simulink model "Appl_PowerMangeModel"  (R2018b)
settings: configuration reference "CodeConfig_10_ms" (kept outside this file)
undefined symbols (not defined in the file): CAL_DownVolt_600ms, CAL_Filiter_500ms, CAL_UpVolt_200ms, D_POWER_ADJUST_15800MV, D_POWER_ADJUST_7800MV, D_POWER_HIGH_DN, D_POWER_HIGH_UP, D_POWER_Invalid, D_POWER_LOW_DN, D_POWER_LOW_UP, D_POWER_NORMAL_DN, D_POWER_NORMAL_UP, D_POWER_OVER_DN, D_POWER_STOP_UP, enPowerModeSts, FALSE, TRUE
libraries: DareLib x7, simulink x5
settings Model: Creator=Administrator  LastModifiedBy=Administrator
settings ConfigSetRef: SourceLocation=Base Workspace

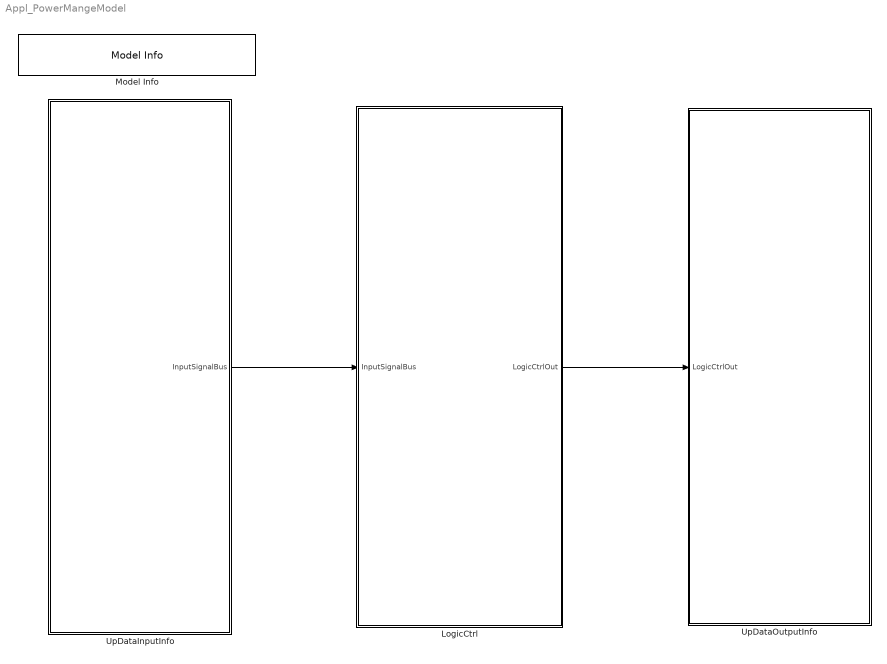
== system Appl_PowerMangeModel ==
  LogicCtrl : Subsystem  Priority=2  TreatAsAtomicUnit=on
      settings: RTWSystemCode=Nonreusable function  RTWFcnNameOpts=Use subsystem name
  Model Info : simulink/Model-Wide Utilities/Model Info  Frame=on  DisplayStringWithTags=Version：%<ModelVersion>  HorizontalTextAlignment=Center  LeftAlignmentValue=0.5
  UpDataInputInfo : Subsystem  Priority=1  TreatAsAtomicUnit=on
      settings: RTWSystemCode=Nonreusable function  RTWFcnNameOpts=Use subsystem name
  UpDataOutputInfo : Subsystem  Priority=3  TreatAsAtomicUnit=on
      settings: RTWSystemCode=Nonreusable function  RTWFcnNameOpts=Use subsystem name
  wires:
  UpDataInputInfo/1(InputSignalBus) -> LogicCtrl/1(InputSignalBus)
  LogicCtrl/1(LogicCtrlOut) -> UpDataOutputInfo/1(LogicCtrlOut)

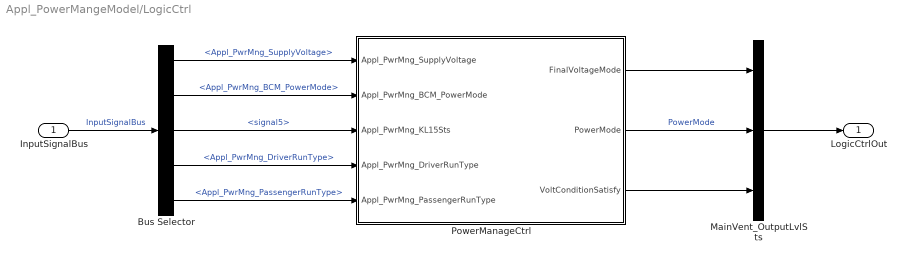
== system Appl_PowerMangeModel/LogicCtrl ==
  InputSignalBus : Inport
  Bus Selector : BusSelector  OutputSignals=Rte_SignalBus.Appl_PwrMng_SupplyVoltage,Rte_SignalBus.Appl_PwrMng_BCM_PowerMode,Rte_SignalBus.signal5,Rte_SignalBus.Appl_PwrMng_DriverRunType,Rte_SignalBus.Appl_PwrMng_PassengerRunType
  MainVent_OutputLvlSts : BusCreator  Inputs=3
  PowerManageCtrl : Subsystem  Description=电源管理逻辑处理
      settings: AttributesFormatString=%<Description>
  LogicCtrlOut : Outport
  wires:
  InputSignalBus/1 -> Bus Selector/1  "InputSignalBus"
  MainVent_OutputLvlSts/1 -> LogicCtrlOut/1
  PowerManageCtrl/1(FinalVoltageMode) -> MainVent_OutputLvlSts/1
  Bus Selector/2 -> PowerManageCtrl/2(Appl_PwrMng_BCM_PowerMode)  "<Appl_PwrMng_BCM_PowerMode>"
  Bus Selector/1 -> PowerManageCtrl/1(Appl_PwrMng_SupplyVoltage)  "<Appl_PwrMng_SupplyVoltage>"
  Bus Selector/3 -> PowerManageCtrl/3(Appl_PwrMng_KL15Sts)  "<signal5>"
  PowerManageCtrl/2(PowerMode) -> MainVent_OutputLvlSts/2  "PowerMode"
  Bus Selector/4 -> PowerManageCtrl/4(Appl_PwrMng_DriverRunType)  "<Appl_PwrMng_DriverRunType>"
  Bus Selector/5 -> PowerManageCtrl/5(Appl_PwrMng_PassengerRunType)  "<Appl_PwrMng_PassengerRunType>"
  PowerManageCtrl/3(VoltConditionSatisfy) -> MainVent_OutputLvlSts/3

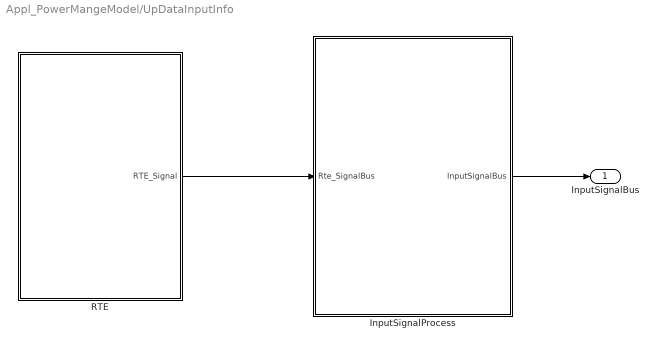
== system Appl_PowerMangeModel/UpDataInputInfo ==
  InputSignalProcess : Subsystem  Description=数据处理
      settings: AttributesFormatString=%<Description>  RTWSystemCode=Nonreusable function  RTWFcnNameOpts=Use subsystem name
  RTE : Subsystem  Description=接口自动生成  TreatAsAtomicUnit=on
      settings: AttributesFormatString=%<Description>  RTWSystemCode=Nonreusable function  RTWFcnNameOpts=Use subsystem name
  InputSignalBus : Outport
  wires:
  RTE/1(RTE_Signal) -> InputSignalProcess/1(Rte_SignalBus)
  InputSignalProcess/1(InputSignalBus) -> InputSignalBus/1

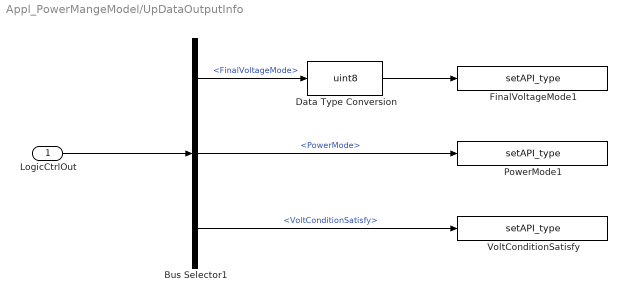
== system Appl_PowerMangeModel/UpDataOutputInfo ==
  LogicCtrlOut : Inport
  Bus Selector1 : BusSelector  OutputSignals=FinalVoltageMode,PowerMode,VoltConditionSatisfy
  Data Type Conversion : DataTypeConversion  OutDataTypeStr=uint8
  FinalVoltageMode1 : DareLib/Dare/setAPI_type  g_funcname=Rte_SetVfb_VoltMode  g_type=uint8  g_size=-1
      settings: AttributesFormatString=%<g_funcname>  SourceProductName=Dare Library
  PowerMode1 : DareLib/Dare/setAPI_type  g_funcname=Rte_SetVfb_PowerMode  g_type=uint8  g_size=-1
      settings: AttributesFormatString=%<g_funcname>  SourceProductName=Dare Library
  VoltConditionSatisfy : DareLib/Dare/setAPI_type  g_funcname=Rte_SetVfb_VoltSatisfy  g_type=uint8  g_size=-1
      settings: AttributesFormatString=%<g_funcname>  SourceProductName=Dare Library
  wires:
  LogicCtrlOut/1 -> Bus Selector1/1
  Bus Selector1/1 -> Data Type Conversion/1  "<FinalVoltageMode>"
  Bus Selector1/2 -> PowerMode1/1  "<PowerMode>"
  Data Type Conversion/1 -> FinalVoltageMode1/1
  Bus Selector1/3 -> VoltConditionSatisfy/1  "<VoltConditionSatisfy>"

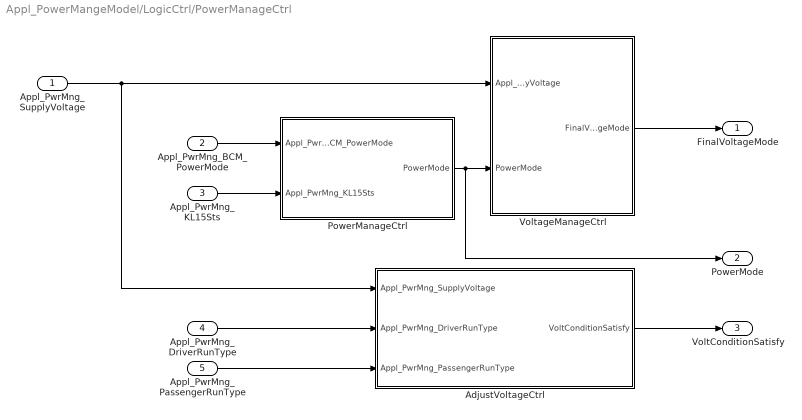
== system Appl_PowerMangeModel/LogicCtrl/PowerManageCtrl ==
  Appl_PwrMng_SupplyVoltage : Inport
  Appl_PwrMng_BCM_PowerMode : Inport  Port=2
  Appl_PwrMng_KL15Sts : Inport  Port=3
  Appl_PwrMng_DriverRunType : Inport  Port=4
  Appl_PwrMng_PassengerRunType : Inport  Port=5
  AdjustVoltageCtrl : Subsystem  Description=调节电机电压控制
      settings: AttributesFormatString=%<Description>
  PowerManageCtrl : Subsystem  Description=系统电源模式管理
      settings: AttributesFormatString=%<Description>
  VoltageManageCtrl : Subsystem  Description=电压模式切换
      settings: AttributesFormatString=%<Description>
  FinalVoltageMode : Outport
  PowerMode : Outport  Port=2
  VoltConditionSatisfy : Outport  Port=3
  wires:
  VoltageManageCtrl/1(FinalVoltageMode) -> FinalVoltageMode/1
  Appl_PwrMng_SupplyVoltage/1 -> AdjustVoltageCtrl/1(Appl_PwrMng_SupplyVoltage), VoltageManageCtrl/1(Appl_PwrMng_SupplyVoltage)
  Appl_PwrMng_KL15Sts/1 -> PowerManageCtrl/2(Appl_PwrMng_KL15Sts)
  PowerManageCtrl/1(PowerMode) -> PowerMode/1, VoltageManageCtrl/2(PowerMode)
  Appl_PwrMng_BCM_PowerMode/1 -> PowerManageCtrl/1(Appl_PwrMng_BCM_PowerMode)
  Appl_PwrMng_DriverRunType/1 -> AdjustVoltageCtrl/2(Appl_PwrMng_DriverRunType)
  Appl_PwrMng_PassengerRunType/1 -> AdjustVoltageCtrl/3(Appl_PwrMng_PassengerRunType)
  AdjustVoltageCtrl/1(VoltConditionSatisfy) -> VoltConditionSatisfy/1

== system Appl_PowerMangeModel/UpDataInputInfo/InputSignalProcess ==
  Rte_SignalBus : Inport
  Bus Creator : BusCreator  Inputs=1
  InputSignalBus : Outport
  wires:
  Bus Creator/1 -> InputSignalBus/1
  Rte_SignalBus/1 -> Bus Creator/1  "Rte_SignalBus"

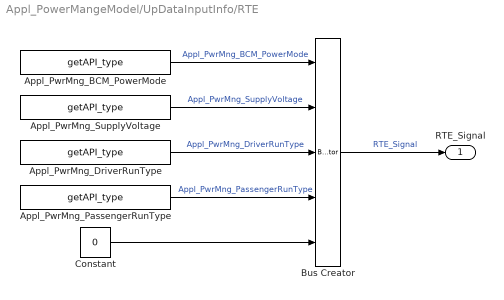
== system Appl_PowerMangeModel/UpDataInputInfo/RTE ==
  Appl_PwrMng_BCM_PowerMode : DareLib/Dare/getAPI_type  g_funcname=CanRx_0x283_BDC_PDU  g_param=""  g_type=uint8  g_size=-1
      settings: AttributesFormatString=%<g_funcname>  SourceProductName=Dare Library
  Appl_PwrMng_DriverRunType : DareLib/Dare/getAPI_type  g_funcname=Rte_GetVfb_DrMoveType  g_param=""  g_type=uint8  g_enum=enSeatMotorRunTye  g_size=-1
      settings: AttributesFormatString=%<g_funcname>  SourceProductName=Dare Library
  Appl_PwrMng_PassengerRunType : DareLib/Dare/getAPI_type  g_funcname=Rte_GetVfb_PaMoveType  g_param=""  g_type=uint8  g_enum=enSeatMotorRunTye  g_size=-1
      settings: AttributesFormatString=%<g_funcname>  SourceProductName=Dare Library
  Appl_PwrMng_SupplyVoltage : DareLib/Dare/getAPI_type  g_funcname=Srvl_Get_SupplyVoltage  g_param=""  g_type=uint16  g_size=-1
      settings: AttributesFormatString=%<g_funcname>  SourceProductName=Dare Library
  Bus Creator : BusCreator  Inputs=5
  Constant : Constant  Value=0  OutDataTypeStr=uint8
  RTE_Signal : Outport
  wires:
  Bus Creator/1 -> RTE_Signal/1  "RTE_Signal"
  Appl_PwrMng_BCM_PowerMode/1 -> Bus Creator/1  "Appl_PwrMng_BCM_PowerMode"
  Appl_PwrMng_SupplyVoltage/1 -> Bus Creator/2  "Appl_PwrMng_SupplyVoltage"
  Appl_PwrMng_DriverRunType/1 -> Bus Creator/3  "Appl_PwrMng_DriverRunType"
  Appl_PwrMng_PassengerRunType/1 -> Bus Creator/4  "Appl_PwrMng_PassengerRunType"
  Constant/1 -> Bus Creator/5

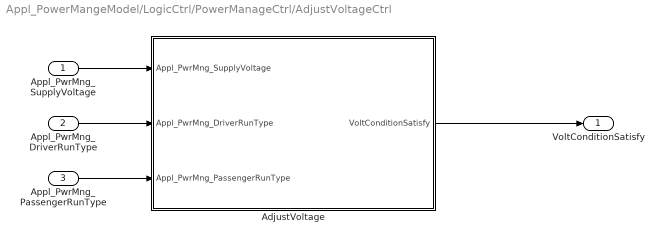
== system Appl_PowerMangeModel/LogicCtrl/PowerManageCtrl/AdjustVoltageCtrl ==
  Appl_PwrMng_SupplyVoltage : Inport
  Appl_PwrMng_DriverRunType : Inport  Port=2
  Appl_PwrMng_PassengerRunType : Inport  Port=3
  AdjustVoltage : Stateflow chart  TreatAsAtomicUnit=on
  VoltConditionSatisfy : Outport
  wires:
  Appl_PwrMng_SupplyVoltage/1 -> AdjustVoltage/1(Appl_PwrMng_SupplyVoltage)
  AdjustVoltage/1(VoltConditionSatisfy) -> VoltConditionSatisfy/1
  Appl_PwrMng_DriverRunType/1 -> AdjustVoltage/2(Appl_PwrMng_DriverRunType)
  Appl_PwrMng_PassengerRunType/1 -> AdjustVoltage/3(Appl_PwrMng_PassengerRunType)

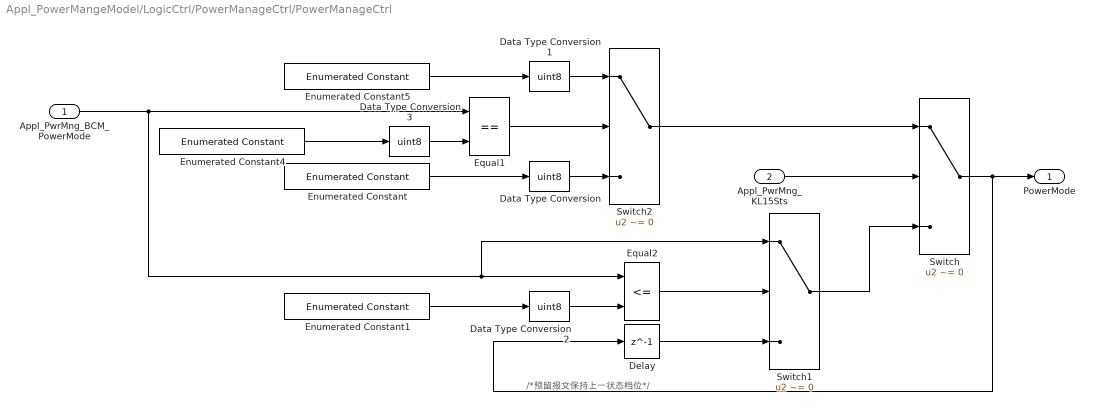
== system Appl_PowerMangeModel/LogicCtrl/PowerManageCtrl/PowerManageCtrl ==
  note: /*预留报文保持上一状态档位*/
  Appl_PwrMng_BCM_PowerMode : Inport
  Appl_PwrMng_KL15Sts : Inport  Port=2
  Data Type Conversion{,1..3} (4 alike) : DataTypeConversion  OutDataTypeStr=uint8
  Delay : Delay  DelayLength=1  InitialCondition=0  InputProcessing=Inherited
  Enumerated Constant : simulink/Sources/Enumerated Constant  OutDataTypeStr=Enum: enPowerModeSts  Value=enPowerModeSts.EN_ON  SampleTime=inf
      settings: SourceProductName=Simulink
  Enumerated Constant1 : simulink/Sources/Enumerated Constant  OutDataTypeStr=Enum: enPowerModeSts  Value=enPowerModeSts.EN_CRANK  SampleTime=inf
      settings: SourceProductName=Simulink
  Enumerated Constant4 : simulink/Sources/Enumerated Constant  OutDataTypeStr=Enum: enPowerModeSts  Value=enPowerModeSts.EN_CRANK  SampleTime=inf
      settings: SourceProductName=Simulink
  Enumerated Constant5 : simulink/Sources/Enumerated Constant  OutDataTypeStr=Enum: enPowerModeSts  Value=enPowerModeSts.EN_CRANK  SampleTime=inf
      settings: SourceProductName=Simulink
  Equal1 : RelationalOperator  Operator===  OutDataTypeStr=boolean  RndMeth=Simplest
  Equal2 : RelationalOperator  Operator=<=  OutDataTypeStr=boolean  RndMeth=Simplest
  Switch : Switch  Criteria=u2 ~= 0
  Switch1 : Switch  Criteria=u2 ~= 0  OutDataTypeStr=uint8
  Switch2 : Switch  Criteria=u2 ~= 0  OutDataTypeStr=uint8
  PowerMode : Outport
  wires:
  Appl_PwrMng_KL15Sts/1 -> Switch/2
  Enumerated Constant/1 -> Data Type Conversion/1
  Enumerated Constant4/1 -> Data Type Conversion3/1
  Equal1/1 -> Switch2/2
  Enumerated Constant5/1 -> Data Type Conversion1/1
  Switch2/1 -> Switch/1
  Enumerated Constant1/1 -> Data Type Conversion2/1
  Appl_PwrMng_BCM_PowerMode/1 -> Switch1/1, Equal2/1, Equal1/1
  Equal2/1 -> Switch1/2
  Switch1/1 -> Switch/3
  Delay/1 -> Switch1/3
  Switch/1 -> Delay/1, PowerMode/1
  Data Type Conversion/1 -> Switch2/3
  Data Type Conversion1/1 -> Switch2/1
  Data Type Conversion2/1 -> Equal2/2
  Data Type Conversion3/1 -> Equal1/2

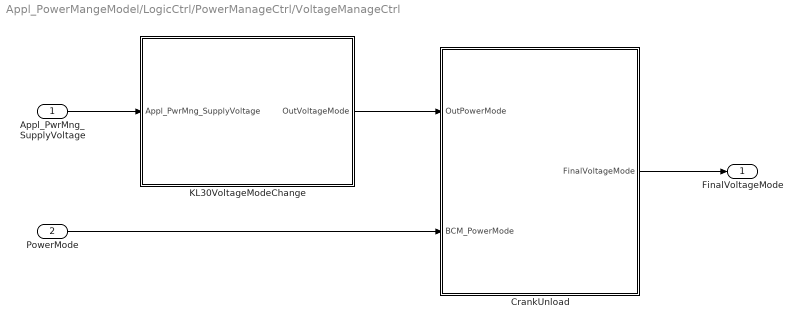
== system Appl_PowerMangeModel/LogicCtrl/PowerManageCtrl/VoltageManageCtrl ==
  Appl_PwrMng_SupplyVoltage : Inport
  PowerMode : Inport  Port=2
  CrankUnload : Stateflow chart  TreatAsAtomicUnit=on
  KL30VoltageModeChange : Stateflow chart  TreatAsAtomicUnit=on
  FinalVoltageMode : Outport
  wires:
  CrankUnload/1(FinalVoltageMode) -> FinalVoltageMode/1
  Appl_PwrMng_SupplyVoltage/1 -> KL30VoltageModeChange/1(Appl_PwrMng_SupplyVoltage)
  PowerMode/1 -> CrankUnload/2(BCM_PowerMode)
  KL30VoltageModeChange/1(OutVoltageMode) -> CrankUnload/1(OutPowerMode)

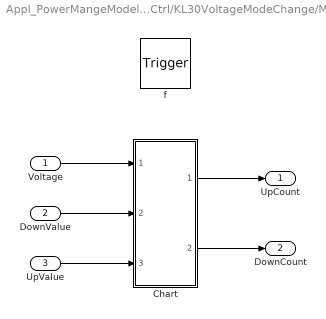
== system Appl_PowerMangeModel/LogicCtrl/PowerManageCtrl/VoltageManageCtrl/KL30VoltageModeChange/ModeChangeFunction ==
  Voltage : Inport  OutDataTypeStr=uint16
  DownValue : Inport  Port=2  OutDataTypeStr=uint16
  UpValue : Inport  Port=3  OutDataTypeStr=uint16
  f : TriggerPort  TriggerType=function-call  VariantControl=(inherit)
      settings: CopyFcn=Stateflow.SLINSF.SimulinkMan.removeBlockPreDeleteFcn  PreDeleteFcn=Stateflow.SLINSF.SimulinkMan.unsafePredeleteFcn
  Chart : Stateflow chart  TreatAsAtomicUnit=on
  UpCount : Outport
  DownCount : Outport  Port=2
  wires:
  Voltage/1 -> Chart/1(Voltage)
  DownValue/1 -> Chart/2(DownValue)
  Chart/1(UpCount) -> UpCount/1
  UpValue/1 -> Chart/3(UpValue)
  Chart/2(DownCount) -> DownCount/1

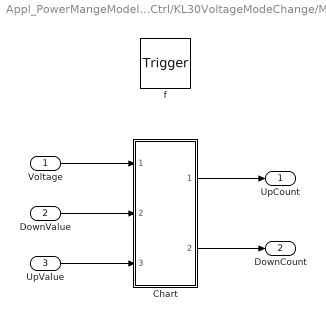
== system Appl_PowerMangeModel/LogicCtrl/PowerManageCtrl/VoltageManageCtrl/KL30VoltageModeChange/ModeChangeFunction1 ==
  Voltage : Inport  OutDataTypeStr=uint16
  DownValue : Inport  Port=2  OutDataTypeStr=uint16
  UpValue : Inport  Port=3  OutDataTypeStr=uint16
  f : TriggerPort  TriggerType=function-call  VariantControl=(inherit)
      settings: CopyFcn=Stateflow.SLINSF.SimulinkMan.removeBlockPreDeleteFcn  PreDeleteFcn=Stateflow.SLINSF.SimulinkMan.unsafePredeleteFcn
  Chart : Stateflow chart  TreatAsAtomicUnit=on
  UpCount : Outport
  DownCount : Outport  Port=2
  wires:
  Voltage/1 -> Chart/1(Voltage)
  DownValue/1 -> Chart/2(DownValue)
  Chart/1(UpCount) -> UpCount/1
  UpValue/1 -> Chart/3(UpValue)
  Chart/2(DownCount) -> DownCount/1

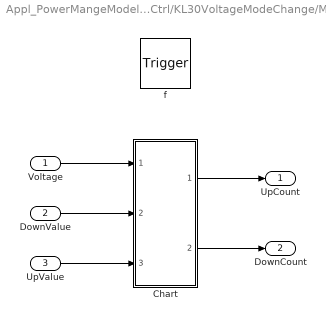
== system Appl_PowerMangeModel/LogicCtrl/PowerManageCtrl/VoltageManageCtrl/KL30VoltageModeChange/ModeChangeFunction2 ==
  Voltage : Inport  OutDataTypeStr=uint16
  DownValue : Inport  Port=2  OutDataTypeStr=uint16
  UpValue : Inport  Port=3  OutDataTypeStr=uint16
  f : TriggerPort  TriggerType=function-call  VariantControl=(inherit)
      settings: CopyFcn=Stateflow.SLINSF.SimulinkMan.removeBlockPreDeleteFcn  PreDeleteFcn=Stateflow.SLINSF.SimulinkMan.unsafePredeleteFcn
  Chart : Stateflow chart  TreatAsAtomicUnit=on
  UpCount : Outport
  DownCount : Outport  Port=2
  wires:
  Voltage/1 -> Chart/1(Voltage)
  DownValue/1 -> Chart/2(DownValue)
  Chart/1(UpCount) -> UpCount/1
  UpValue/1 -> Chart/3(UpValue)
  Chart/2(DownCount) -> DownCount/1

== stateflow chart Appl_PowerMangeModel/LogicCtrl/PowerManageCtrl/VoltageManageCtrl/KL30VoltageModeChange/ModeChangeFunction1/Chart ==
  state VoltDownWait
    en:
    UpCount = 0;
    du:
    DownCount ++;
  state Init
    en:
    UpCount = 1;
    DownCount = 1;
  state VoltUpWait
    en:
    DownCount = 0;
    du:
    UpCount ++;
  (default) -> Init
  Init -> VoltDownWait [order 1] : [Voltage < DownValue]
  Init -> VoltUpWait [order 2] : [Voltage > UpValue]
  VoltDownWait -> Init : [Voltage >= DownValue]
  VoltUpWait -> Init : [Voltage  <= UpValue]
  data: Voltage input; DownValue input; UpValue input; UpCount output uint16; DownCount output uint16

== stateflow chart Appl_PowerMangeModel/LogicCtrl/PowerManageCtrl/VoltageManageCtrl/KL30VoltageModeChange/ModeChangeFunction2/Chart ==
  state VoltDownWait
    en:
    UpCount = 0;
    du:
    DownCount ++;
  state Init
    en:
    UpCount = 1;
    DownCount = 1;
  state VoltUpWait
    en:
    DownCount = 0;
    du:
    UpCount ++;
  (default) -> Init
  Init -> VoltDownWait [order 1] : [Voltage < DownValue]
  Init -> VoltUpWait [order 2] : [Voltage > UpValue]
  VoltDownWait -> Init : [Voltage >= DownValue]
  VoltUpWait -> Init : [Voltage  <= UpValue]
  data: Voltage input; DownValue input; UpValue input; UpCount output uint16; DownCount output uint16

== stateflow chart Appl_PowerMangeModel/LogicCtrl/PowerManageCtrl/AdjustVoltageCtrl/AdjustVoltage ==
  state VoltageSatisfyProcess [parallel]
    settings: executionOrder=1
    (default) -> (junction 19)
    VoltageSatisfyProcess -> (junction 19)
    (junction 19) -> (junction 22) [order 1] : /*电压＞16V*/
        | [D_POWER_HIGH_DN < Appl_PwrMng_SupplyVoltage]
    (junction 19) -> (junction 26) [order 2]
    (junction 22) -> (junction 24) : {StaticVoltageOKFlag = D_POWER_Invalid;}
    (junction 26) -> (junction 28) [order 1] : /*电压 <= 15.8V（高压回差0.2V）*/
        | [D_POWER_ADJUST_15800MV >= Appl_PwrMng_SupplyVoltage]
    (junction 26) -> (junction 32) [order 2]
    (junction 28) -> (junction 30) : {StaticVoltageOKFlag = FALSE;}
    (junction 30) -> (junction 32)
    (junction 24) -> (junction 30)
    (junction 32) -> (junction 142)
    (junction 142) -> (junction 143) [order 1] : /*电压由高压回到正常范围，或者处在正常范围(9V~16V)*/
        | [D_POWER_LOW_UP <= Appl_PwrMng_SupplyVoltage && D_POWER_HIGH_DN >= Appl_PwrMng_SupplyVoltage ...
        | && FALSE == StaticVoltageOKFlag]
    (junction 142) -> (junction 145) [order 2]
    (junction 143) -> (junction 147) : {StaticVoltageOKFlag = TRUE;}
    (junction 147) -> (junction 145)
    (junction 145) -> (junction 36)
    (junction 36) -> (junction 62) [order 1] : /*电压< 7.8V || 电压 >16V（低回差1.2V，避免低压继电器无法吸合问题）NXP及芯旺微*/
        | [D_POWER_ADJUST_7800MV > Appl_PwrMng_SupplyVoltage || D_POWER_HIGH_DN < Appl_PwrMng_SupplyVoltage]
    (junction 36) -> (junction 66) [order 2] : {RunVoltageOKFlag = TRUE;}
    (junction 62) -> (junction 64) : {RunVoltageOKFlag = FALSE;}
    (junction 64) -> (junction 66)
    (junction 66) -> (junction 69)
  state AcquireVoltage [parallel]
    settings: executionOrder=2
    state Default
      en:
      NomalCnt = 0;
      (default) -> (junction 39)
      Default -> (junction 39) [order 1]
      (junction 39) -> (junction 42) [order 1] : /*未初始化过*/
          | [FALSE == InitFlag]
      (junction 39) -> (junction 46) [order 2]
      (junction 42) -> (junction 44) : {InitFlag = TRUE;
          | VoltConditionSatisfy = TRUE;}
      (junction 44) -> (junction 46)
      (junction 46) -> (junction 131)
      (junction 131) -> (junction 132) [order 1] : [AbnomalCnt < CAL_Filiter_500ms]
      (junction 131) -> (junction 133) [order 2] : {AbnomalCnt = CAL_Filiter_500ms;}
      (junction 132) -> (junction 134) : {AbnomalCnt ++;}
      (junction 134) -> (junction 133)
      (junction 133) -> (junction 135)
    state VoltageChecking
      state NormalCounting
        en:
        AbnomalCnt = 0;
        (default) -> (junction 89)
        NormalCounting -> (junction 89) [order 1]
        (junction 89) -> (junction 87) [order 1] : [NomalCnt < CAL_Filiter_500ms]
        (junction 89) -> (junction 82) [order 2] : {NomalCnt = CAL_Filiter_500ms;}
        (junction 87) -> (junction 81) : {NomalCnt ++;}
        (junction 81) -> (junction 82)
        (junction 82) -> (junction 84)
      state AbnormalCounting
        en:
        NomalCnt = 0;
        (default) -> (junction 57)
        AbnormalCounting -> (junction 57) [order 1]
        (junction 57) -> (junction 60) [order 1] : [AbnomalCnt < CAL_Filiter_500ms]
        (junction 57) -> (junction 74) [order 2] : {AbnomalCnt = CAL_Filiter_500ms;}
        (junction 60) -> (junction 72) : {AbnomalCnt ++;}
        (junction 72) -> (junction 74)
        (junction 74) -> (junction 77)
      AbnormalCounting -> NormalCounting [order 1] : /*电机静止电压条件满足9V~16V*/
          | [TRUE == StaticVoltageOKFlag]
      NormalCounting -> AbnormalCounting [order 1] : /*电机调节中，需要注意电压回差，避免无法堵转*/
          | [(enSeatMotorRunTye.EN_NULL != Appl_PwrMng_DriverRunType ...
          | || enSeatMotorRunTye.EN_NULL != Appl_PwrMng_PassengerRunType) ...
          | && TRUE != RunVoltageOKFlag]
    (default) -> Default
    Default -> AbnormalCounting [order 1] : /*电机调节中，需要注意电压回差，避免无法堵转*/
        | [(enSeatMotorRunTye.EN_NULL != Appl_PwrMng_DriverRunType ...
        | || enSeatMotorRunTye.EN_NULL != Appl_PwrMng_PassengerRunType) ...
        | && TRUE != RunVoltageOKFlag]
    VoltageChecking -> Default : /*无主副驾调节请求 && (运动电压不满足8.9V~16V || 电机静止电压不满足9V~16V)*/
        | [(enSeatMotorRunTye.EN_NULL == Appl_PwrMng_DriverRunType ...
        | && enSeatMotorRunTye.EN_NULL == Appl_PwrMng_PassengerRunType) ...
        | && (TRUE != StaticVoltageOKFlag || TRUE != RunVoltageOKFlag)]
    Default -> NormalCounting [order 2] : /*电机静止电压条件满足9V~16V*/
        | [TRUE == StaticVoltageOKFlag]
  state VoltageCheckResult [parallel]
    settings: executionOrder=3
    (default) -> (junction 92)
    VoltageCheckResult -> (junction 92)
    (junction 92) -> (junction 95) [order 1] : /*电压异常滤波时间到*/
        | [CAL_Filiter_500ms <= AbnomalCnt ]
    (junction 92) -> (junction 99) [order 2]
    (junction 95) -> (junction 97) : {VoltConditionSatisfy = FALSE;}
    (junction 97) -> (junction 99)
    (junction 99) -> (junction 102)
    (junction 102) -> (junction 104) [order 1] : /*电压正常滤波时间到*/
        | [CAL_Filiter_500ms <= NomalCnt ]
    (junction 102) -> (junction 108) [order 2]
    (junction 104) -> (junction 106) : {VoltConditionSatisfy = TRUE;}
    (junction 106) -> (junction 108)
    (junction 108) -> (junction 111)
  data: Appl_PwrMng_SupplyVoltage input; Appl_PwrMng_DriverRunType input; Appl_PwrMng_PassengerRunType input; VoltConditionSatisfy output uint8; D_POWER_ADJUST_7800MV parameter; D_POWER_ADJUST_15800MV parameter; InitFlag local uint8 =0; AbnomalCnt local uint8; NomalCnt local uint8; StaticVoltageOKFlag local uint8; RunVoltageOKFlag local uint8; TRUE parameter; FALSE parameter; D_POWER_HIGH_DN parameter; D_POWER_LOW_UP parameter; CAL_Filiter_500ms parameter; D_POWER_Invalid parameter

== stateflow chart Appl_PowerMangeModel/LogicCtrl/PowerManageCtrl/VoltageManageCtrl/CrankUnload ==
  settings: description=卸荷
  state Init
    du:
    FinalVoltageMode = OutPowerMode;
    TempPowerMode = OutPowerMode;
  state CRANK
    du:
    FinalVoltageMode = TempPowerMode;
  (default) -> Init
  CRANK -> Init : [BCM_PowerMode != ...
      | enPowerModeSts.EN_CRANK]
  Init -> CRANK : [BCM_PowerMode == ...
      | enPowerModeSts.EN_CRANK]
  data: OutPowerMode input; FinalVoltageMode output Enum: enFinalPowerMode; BCM_PowerMode input; TempPowerMode local Enum: enFinalPowerMode

== stateflow chart Appl_PowerMangeModel/LogicCtrl/PowerManageCtrl/VoltageManageCtrl/KL30VoltageModeChange ==
  settings: description=蓄电池电源模式切换
  state [UpCount,DownCount] = ModeChangeFunction(Voltage,DownValue,UpValue) [function]
  state [UpCount,DownCount] = ModeChangeFunction1(Voltage,DownValue,UpValue) [function]
  state [UpCount,DownCount] = ModeChangeFunction2(Voltage,DownValue,UpValue) [function]
  state BelowNormal
    state Stop
      en:
      OutVoltageMode = enFinalPowerMode.EN_STOP_VOLT;/*0=停止模式*/
      ex:
      UpTimer = 0;
      (default) -> (junction 116)
      Stop -> (junction 116) [order 1]
      (junction 116) -> (junction 124) [order 1] : /*系统电压>停止模式上限电压*/
          | [Appl_PwrMng_SupplyVoltage > D_POWER_STOP_UP]
      (junction 116) -> (junction 128) [order 2] : /*系统电压<=停止模式上限电压*/
          | {UpTimer = 0;
          | OutVoltageMode = enFinalPowerMode.EN_STOP_VOLT;}
      (junction 124) -> (junction 130) : {UpTimer ++;}
      (junction 130) -> (junction 128)
      (junction 128) -> (junction 215)
    state Low
      en:
      OutVoltageMode = enFinalPowerMode.EN_LOW_VOLT;/*1=低压模式*/
      du:
      [UpTimer,DownTimer] = ModeChangeFunction(Appl_PwrMng_SupplyVoltage, D_POWER_LOW_DN, D_POWER_LOW_UP);
      ex:
      UpTimer = 0;
      DownTimer = 0;
    (junction 177) -> Stop [order 1] : /*系统电压<=低压模式下限*/
        | [Appl_PwrMng_SupplyVoltage ...
        | <= D_POWER_LOW_DN]
    Low -> Stop : /*系统电压<电压模式下限持续600ms*/
        | [DownTimer >= CAL_DownVolt_600ms]
    Stop -> Low [order 1] : /*系统电压>停止模式上限电压*/
        | [UpTimer >= CAL_DownVolt_600ms ...
        | && Appl_PwrMng_SupplyVoltage <= D_POWER_LOW_UP]
    (default) -> (junction 177)
    (junction 177) -> Low [order 2]
  state AboveNormal
    state High
      en:
      OutVoltageMode = enFinalPowerMode.EN_HIGH_VOLT;/*3=高压模式*/
      du:
      [UpTimer,DownTimer] = ModeChangeFunction2(Appl_PwrMng_SupplyVoltage, D_POWER_HIGH_DN, D_POWER_HIGH_UP);
      ex:
      UpTimer = 0;
      DownTimer = 0;
    state Over
      en:
      OutVoltageMode = enFinalPowerMode.EN_OVER_VOLT;/*4=过压模式*/
      ex:
      DownTimer = 0;
      (default) -> (junction 153)
      Over -> (junction 153) [order 1]
      (junction 153) -> (junction 158) [order 1] : /*系统电压<过压模式下限*/
          | [Appl_PwrMng_SupplyVoltage < D_POWER_OVER_DN]
      (junction 153) -> (junction 159) [order 2] : /*系统电压>过压模式上限*/
          | {DownTimer = 0;
          | OutVoltageMode = enFinalPowerMode.EN_OVER_VOLT;}
      (junction 158) -> (junction 155) : {DownTimer  ++;}
      (junction 155) -> (junction 159)
      (junction 159) -> (junction 220)
    (junction 184) -> High [order 2]
    High -> Over : /*系统电压>电压模式上限持续200ms*/
        | [UpTimer >= CAL_UpVolt_200ms]
    Over -> High [order 1] : /*系统电压<电压模式上限持续200ms
        | 且 系统电压>=正常电压上限*/
        | [DownTimer >= CAL_UpVolt_200ms ...
        | && Appl_PwrMng_SupplyVoltage >= D_POWER_NORMAL_UP]
    (default) -> (junction 184)
    (junction 184) -> Over [order 1] : /*系统电压>高压模式上限*/
        | [Appl_PwrMng_SupplyVoltage > D_POWER_HIGH_UP]
  state Normal
    en:
    OutVoltageMode = enFinalPowerMode.EN_NORMAL_VOLT;/*2=正常模式*/
    du:
    [UpTimer,DownTimer] = ModeChangeFunction1(Appl_PwrMng_SupplyVoltage, D_POWER_NORMAL_DN, D_POWER_NORMAL_UP);
    ex:
    UpTimer = 0;
    DownTimer = 0;
  (default) -> Normal
  Normal -> AboveNormal [order 2] : /*在Normal切换到AboveNormal条件：
      | 系统电压>=电压模式上限持续200ms */
      | [UpTimer >= CAL_UpVolt_200ms]
  Normal -> BelowNormal [order 1] : /*在BelowNormal切换到Normal条件：
      | 系统电压<电压模式下限持续600ms*/
      | [DownTimer >= CAL_DownVolt_600ms]
  AboveNormal -> Normal [order 1] : /*在AboveNormal切换到Normal条件：
      | 系统电压>=电压模式上限持续200ms
      | 且 系统电压>=正常电压下限
      | 且 系统电压<正常电压上限*/
      | [DownTimer >= CAL_UpVolt_200ms ...
      | && Appl_PwrMng_SupplyVoltage >= D_POWER_NORMAL_DN ...
      | && Appl_PwrMng_SupplyVoltage < D_POWER_NORMAL_UP]
  BelowNormal -> Normal [order 1] : /*在Normal切换到BelowNormal条件：
      | 系统电压<电压模式上限持续600ms
      | 且 系统电压<正常电压上限
      | 且 系统电压>正常电压下限*/
      | [UpTimer >= CAL_DownVolt_600ms ...
      | && Appl_PwrMng_SupplyVoltage <= D_POWER_NORMAL_UP ...
      | && Appl_PwrMng_SupplyVoltage > D_POWER_LOW_UP]
  BelowNormal -> AboveNormal [order 2] : /*在BelowNormal直接切换到AboveNormal条件：
      | 系统电压>=电压模式上限持续200ms 且 系统电压>正常电压上限*/
      | [UpTimer >= CAL_UpVolt_200ms ...
      | && Appl_PwrMng_SupplyVoltage > D_POWER_NORMAL_UP]
  AboveNormal -> BelowNormal [order 2] : /*在AboveNormal直接切换到BelowNormal条件：
      | 系统电压>=电压模式下限持续600ms 且 系统电压<正常电压下限*/
      | [DownTimer >= CAL_DownVolt_600ms ...
      | && Appl_PwrMng_SupplyVoltage < D_POWER_NORMAL_DN]
  data: Voltage function_input uint16; DownValue function_input uint16; UpCount function_output; UpValue function_input uint16; DownCount function_output; Voltage function_input uint16; DownValue function_input uint16; UpCount function_output; UpValue function_input uint16; DownCount function_output; Voltage function_input uint16; DownValue function_input uint16; UpCount function_output; UpValue function_input uint16; DownCount function_output; Appl_PwrMng_SupplyVoltage input; DownTimer local uint8; UpTimer local uint8; D_POWER_HIGH_DN parameter; D_POWER_HIGH_UP parameter; D_POWER_LOW_DN parameter; D_POWER_LOW_UP parameter; D_POWER_NORMAL_DN parameter; D_POWER_NORMAL_UP parameter; D_POWER_OVER_DN parameter; D_POWER_STOP_UP parameter; CAL_UpVolt_200ms parameter; CAL_DownVolt_600ms parameter; OutVoltageMode output Enum: enFinalPowerMode

== stateflow chart Appl_PowerMangeModel/LogicCtrl/PowerManageCtrl/VoltageManageCtrl/KL30VoltageModeChange/ModeChangeFunction/Chart ==
  state VoltDownWait
    en:
    UpCount = 0;
    du:
    DownCount ++;
  state Init
    en:
    UpCount = 1;
    DownCount = 1;
  state VoltUpWait
    en:
    DownCount = 0;
    du:
    UpCount ++;
  (default) -> Init
  Init -> VoltDownWait [order 1] : [Voltage < DownValue]
  Init -> VoltUpWait [order 2] : [Voltage > UpValue]
  VoltDownWait -> Init : [Voltage >= DownValue]
  VoltUpWait -> Init : [Voltage  <= UpValue]
  data: Voltage input; DownValue input; UpValue input; UpCount output uint16; DownCount output uint16
